simulink model "single_phase_pll_analysis"  (R2025b)
settings: Solver=ode1  StartTime=0.0  StopTime=20  FixedStep=ts_inv  RelTol=1e-3
values from neighbouring files (symbols this model uses):
  Adrso = eye(2) + Arso*ts_afe    [init_model.m]
  Crso = [1 0]    [init_model.m]
  Ldrso = acker(Adrso',Crso',polesdrso)'    [init_model.m]
  omega_set = 2*pi*frequency_set    (= 502.654824574)    [init_model.m]
  ts_inv = tPWM_INV    (= 0.00025)    [init_model.m]
libraries: discrete_time_low_pass_filter x2
settings Model: Creator=dbagn  LastModifiedBy=dbagn

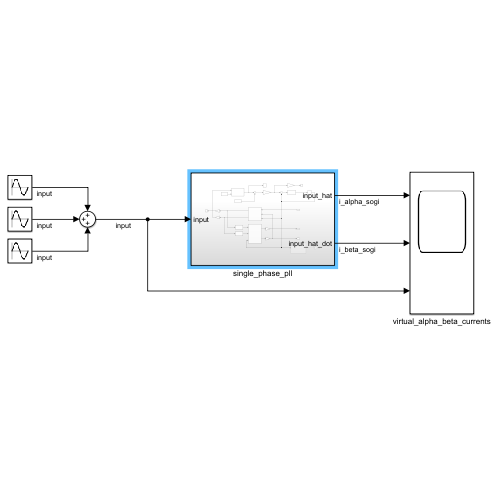
[thumbnail: Simulink's stored preview of the top-level diagram]
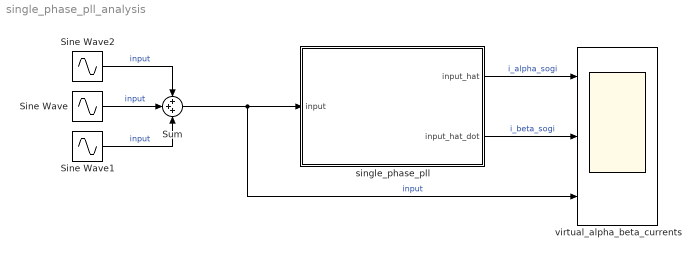
== system single_phase_pll_analysis ==
  Sine Wave : Sin  Frequency=omega_set  Phase=-pi/2  SampleTime=0
  Sine Wave1 : Sin  Amplitude=0.1  Frequency=omega_set*5  SampleTime=0
  Sine Wave2 : Sin  Amplitude=0.1  Frequency=omega_set*11  SampleTime=0
  Sum : Sum  Inputs=+++
  single_phase_pll : Subsystem
  virtual_alpha_beta_currents : Scope  NumInputPorts=3
      settings: ActiveDisplayYMinimum=-1.26517292435703  ActiveDisplayYMaximum=1.2618674614397347  DataLoggingVariableName=ScopeData2
  wires:
  Sum/1 -> single_phase_pll/1(input), virtual_alpha_beta_currents/3  "input"
  single_phase_pll/1(input_hat) -> virtual_alpha_beta_currents/1  "i_alpha_sogi"
  single_phase_pll/2(input_hat_dot) -> virtual_alpha_beta_currents/2  "i_beta_sogi"
  Sine Wave1/1 -> Sum/3  "input"
  Sine Wave/1 -> Sum/2  "input"
  Sine Wave2/1 -> Sum/1  "input"

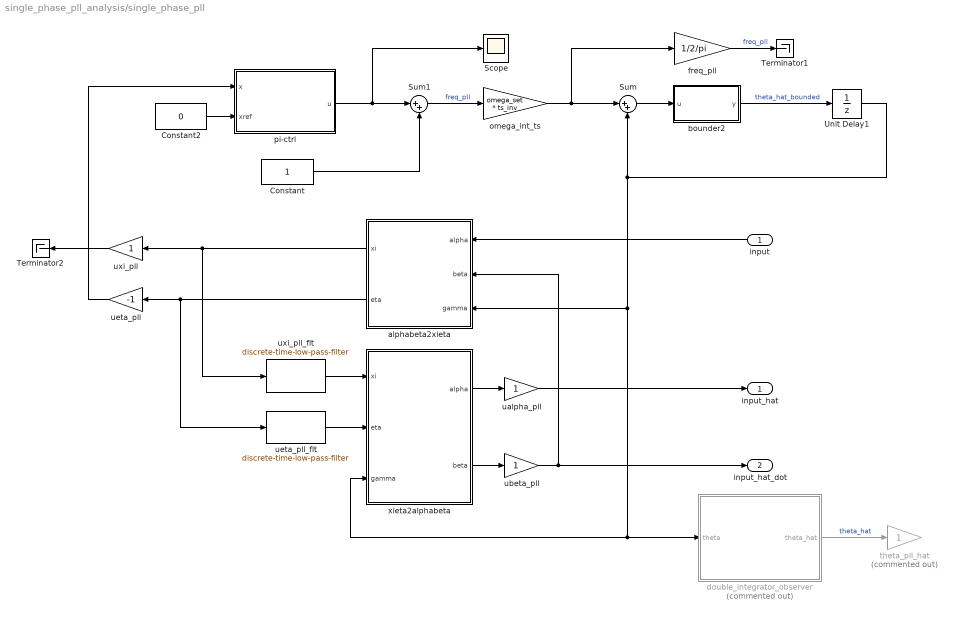
== system single_phase_pll_analysis/single_phase_pll ==
  input : Inport
  Constant : Constant
  Constant2 : Constant  Value=0
  Scope : Scope
      settings: ActiveDisplayYMinimum=-1.1813345026503461  ActiveDisplayYMaximum=0.50653477204197639
  Sum : Sum  Inputs=|++
  Sum1 : Sum  Inputs=|++
  Terminator1 : Terminator
  Terminator2 : Terminator
  Unit Delay1 : UnitDelay  SampleTime=-1  HasFrameUpgradeWarning=on
  alphabeta2xieta : MATLAB Function  TreatAsAtomicUnit=on
  bounder2 : MATLAB Function  TreatAsAtomicUnit=on
  double_integrator_observer : Subsystem  Commented=on
  freq_pll : Gain  Gain=1/2/pi
  omega_int_ts : Gain  Gain=omega_set * ts_inv
  pi-ctrl : Subsystem  mask{kp=1, ki=0, ts=ts_inv, sat_pos=2, sat_neg=-2}
  theta_pll_hat : Gain  Commented=on
  ualpha_pll : Gain
  ubeta_pll : Gain
  ueta_pll : Gain  Gain=-1
  ueta_pll_flt : discrete_time_low_pass_filter/discrete-time-low-pass-filter  tau=2/omega_set  ts=ts_inv
  uxi_pll : Gain
  uxi_pll_flt : discrete_time_low_pass_filter/discrete-time-low-pass-filter  tau=2/omega_set  ts=ts_inv
  xieta2alphabeta : MATLAB Function  TreatAsAtomicUnit=on
  input_hat : Outport
  input_hat_dot : Outport  Port=2
  wires:
  Sum/1 -> bounder2/1(u)
  alphabeta2xieta/1(xi) -> uxi_pll/1, uxi_pll_flt/1
  xieta2alphabeta/2(beta) -> ubeta_pll/1
  alphabeta2xieta/2(eta) -> ueta_pll/1, ueta_pll_flt/1
  omega_int_ts/1 -> freq_pll/1, Sum/1
  double_integrator_observer/1(theta_hat) -> theta_pll_hat/1  "theta_hat"
  input/1 -> alphabeta2xieta/1(alpha)
  freq_pll/1 -> Terminator1/1  "freq_pll"
  ueta_pll_flt/1 -> xieta2alphabeta/2(eta)
  uxi_pll_flt/1 -> xieta2alphabeta/1(xi)
  ueta_pll/1 -> pi-ctrl/1(x)
  Sum1/1 -> omega_int_ts/1  "freq_pll"
  Constant2/1 -> pi-ctrl/2(xref)
  uxi_pll/1 -> Terminator2/1
  ubeta_pll/1 -> alphabeta2xieta/2(beta), input_hat_dot/1
  xieta2alphabeta/1(alpha) -> ualpha_pll/1
  ualpha_pll/1 -> input_hat/1
  pi-ctrl/1(u) -> Sum1/1, Scope/1
  Constant/1 -> Sum1/2
  Unit Delay1/1 -> Sum/2, alphabeta2xieta/3(gamma), xieta2alphabeta/3(gamma), double_integrator_observer/1(theta)
  bounder2/1(y) -> Unit Delay1/1  "theta_hat_bounded"

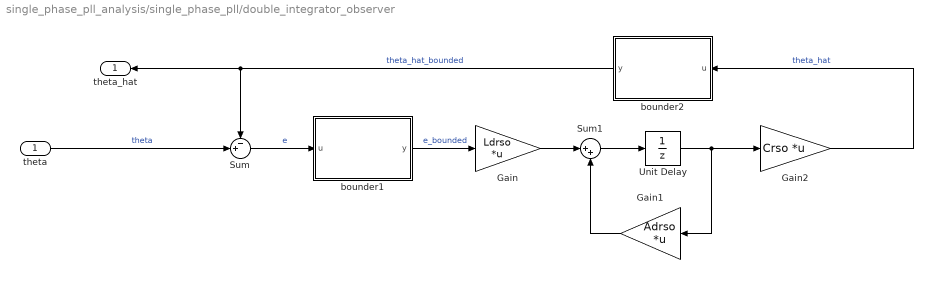
== system single_phase_pll_analysis/single_phase_pll/double_integrator_observer ==
  theta : Inport
  Gain : Gain  Gain=Ldrso  Multiplication=Matrix(K*u)
  Gain1 : Gain  Gain=Adrso  Multiplication=Matrix(K*u)
  Gain2 : Gain  Gain=Crso  Multiplication=Matrix(K*u)
  Sum : Sum  Inputs=-+|
  Sum1 : Sum  Inputs=|++
  Unit Delay : UnitDelay  SampleTime=-1  HasFrameUpgradeWarning=on
  bounder1 : MATLAB Function  TreatAsAtomicUnit=on
  bounder2 : MATLAB Function  TreatAsAtomicUnit=on
  theta_hat : Outport
  wires:
  Gain/1 -> Sum1/1
  Gain2/1 -> bounder2/1(u)  "theta_hat"
  Gain1/1 -> Sum1/2
  Sum1/1 -> Unit Delay/1
  Sum/1 -> bounder1/1(u)  "e"
  Unit Delay/1 -> Gain1/1, Gain2/1
  theta/1 -> Sum/2  "theta"
  bounder1/1(y) -> Gain/1  "e_bounded"
  bounder2/1(y) -> theta_hat/1, Sum/1  "theta_hat_bounded"

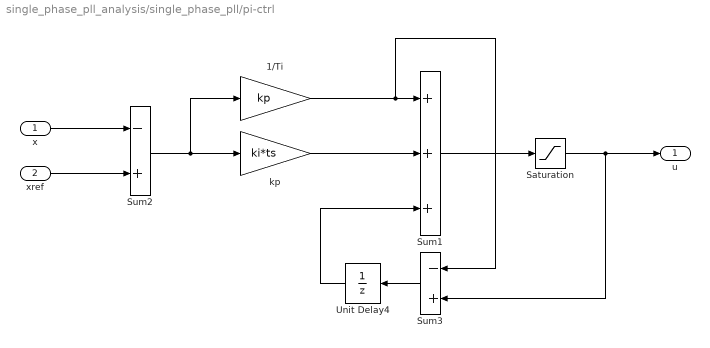
== system single_phase_pll_analysis/single_phase_pll/pi-ctrl ==
  x : Inport
  xref : Inport  Port=2
  1/Ti : Gain  Gain=kp  SaturateOnIntegerOverflow=on  OutDataTypeStr=Inherit: Same as input  ParamDataTypeStr=Inherit: Same as input
  Saturation : Saturate  UpperLimit=sat_pos  LowerLimit=sat_neg
  Sum1 : Sum  Inputs=+++  SaturateOnIntegerOverflow=on
  Sum2 : Sum  Inputs=-+  SaturateOnIntegerOverflow=on
  Sum3 : Sum  Inputs=-+  SaturateOnIntegerOverflow=on
  Unit Delay4 : UnitDelay  SampleTime=-1  HasFrameUpgradeWarning=on
  kp : Gain  Gain=ki*ts  SaturateOnIntegerOverflow=on  OutDataTypeStr=Inherit: Same as input  ParamDataTypeStr=Inherit: Same as input
  u : Outport
  wires:
  Saturation/1 -> Sum3/2, u/1
  Unit Delay4/1 -> Sum1/3
  Sum1/1 -> Saturation/1
  Sum3/1 -> Unit Delay4/1
  1/Ti/1 -> Sum3/1, Sum1/1
  Sum2/1 -> 1/Ti/1, kp/1
  kp/1 -> Sum1/2
  x/1 -> Sum2/1
  xref/1 -> Sum2/2

== matlab function single_phase_pll_analysis/single_phase_pll/alphabeta2xieta ==
  data: alpha input; xi output; beta input; gamma input; eta output
function [xi,eta] = alphabeta2xieta(alpha,beta,gamma)
    xi  =  alpha*cos(gamma) + beta*sin(gamma);
    eta = -alpha*sin(gamma) + beta*cos(gamma);
end

== matlab function single_phase_pll_analysis/single_phase_pll/bounder2 ==
  data: u input; y output
function y = bounder(u)
    
    y = -pi + mod(u+3*pi,2*pi);
   
end

== matlab function single_phase_pll_analysis/single_phase_pll/double_integrator_observer/bounder1 ==
  data: u input; y output
function y = bounder(u)
    
    y = -pi + mod(u+3*pi,2*pi);
   
end

== matlab function single_phase_pll_analysis/single_phase_pll/double_integrator_observer/bounder2 ==
  data: u input; y output
function y = bounder(u)
    
    y = -pi + mod(u+3*pi,2*pi);
   
end

== matlab function single_phase_pll_analysis/single_phase_pll/xieta2alphabeta ==
  data: xi input; alpha output; eta input; gamma input; beta output
function [alpha,beta] = xieta2alphabeta(xi,eta,gamma)
    alpha  = xi*cos(gamma) - eta*sin(gamma);
    beta = xi*sin(gamma) + eta*cos(gamma);
end
